simulink model "static_rod_model_equations"  (R2024b)
settings: Solver=VariableStepAuto  StartTime=0.0  StopTime=30  RelTol=1e-3
settings Model: Creator=utkarsh
settings DataIOCC: SaveFormat=StructureWithTime
settings OptimizationCC: ReuseModelBlockBuffer=off
settings ModelReferenceCC: EnableRefExpFcnMdlSchedulingChecks=on
settings RTWCC: GPUComputeCapability=3.5

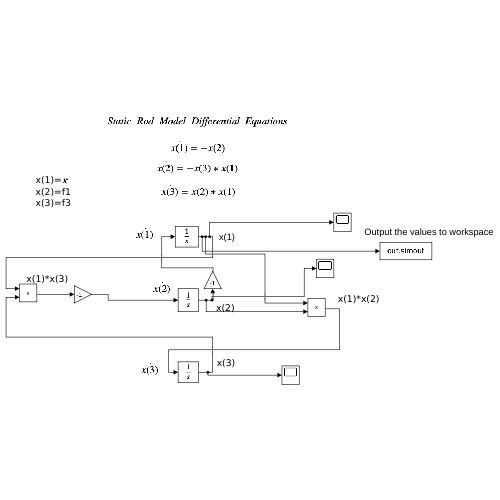
[thumbnail: Simulink's stored preview of the top-level diagram]
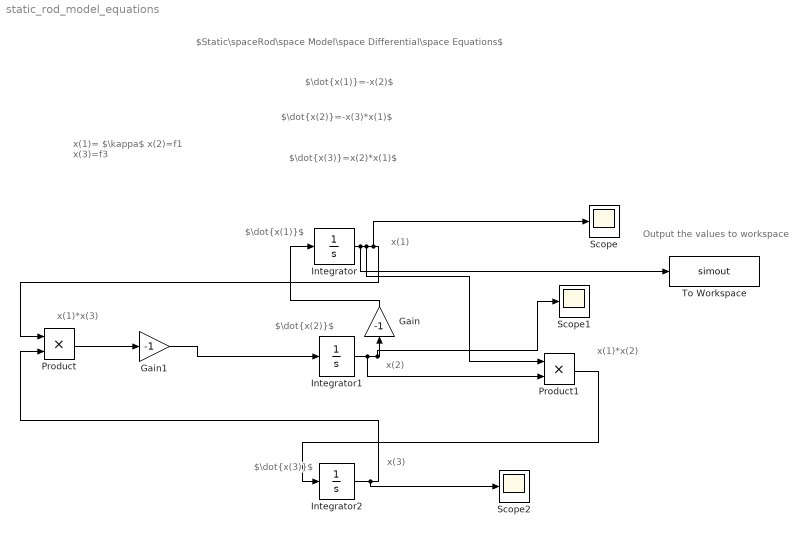
== system static_rod_model_equations ==
  note: x(1)= $\kappa$
      | x(2)=f1
      | x(3)=f3
  note: Output the values to workspace
  note: x(1)*x(2)
  note: x(1)*x(3)
  note: x(3)
  note: x(2)
  note: x(1)
  note: $\dot{x(1)}$
  note: $\dot{x(2)}$
  note: $\dot{x(3)}$
  note: $\dot{x(1)}=-x(2)$
  note: $\dot{x(2)}=-x(3)*x(1)$
  note: $\dot{x(3)}=x(2)*x(1)$
  note: $Static\spaceRod\space Model\space Differential\space Equations$
  Gain : Gain  Gain=-1
  Gain1 : Gain  Gain=-1
  Integrator : Integrator
  Integrator1 : Integrator  InitialCondition=-0.004
  Integrator2 : Integrator
  Product : Product
  Product1 : Product
  Scope : Scope
  Scope1 : Scope
  Scope2 : Scope
  To Workspace : ToWorkspace  VariableName=simout  SaveFormat=Timeseries  SampleTime=-1
  wires:
  Integrator/1 -> To Workspace/1, Product1/1, Scope/1, Product/1
  Integrator1/1 -> Product1/2, Scope1/1, Gain/1
  Gain/1 -> Integrator/1
  Integrator2/1 -> Scope2/1, Product/2
  Product/1 -> Gain1/1
  Gain1/1 -> Integrator1/1
  Product1/1 -> Integrator2/1
